simulink model "mini_project_part21"  (R2023b)
settings: Solver=VariableStepAuto  StartTime=0.0  StopTime=1  RelTol=1e-3
libraries: commdigbbndpm3 x2, commchan3 x1, commrandsrc3 x1, commsink2 x1
settings Model: Creator=lx69  LastModifiedBy=xieluxi

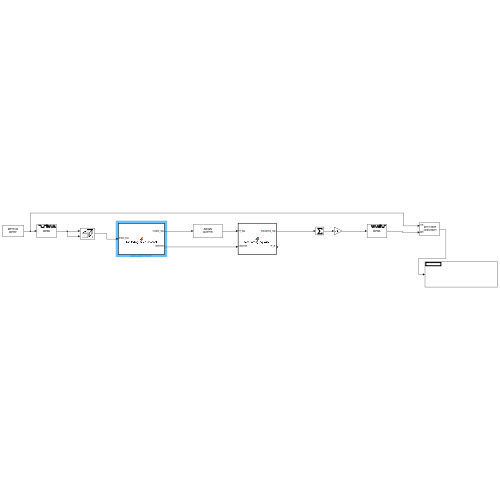
[thumbnail: Simulink's stored preview of the top-level diagram]
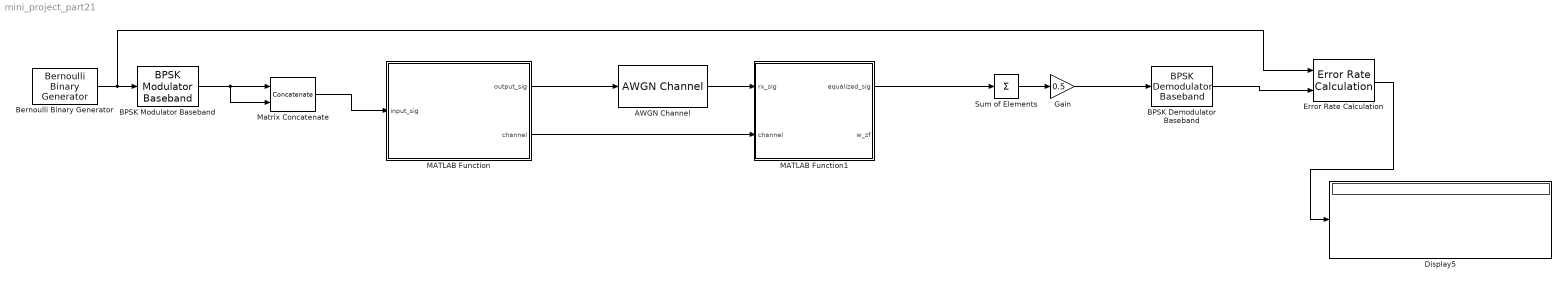
== system mini_project_part21 ==
  AWGN Channel : commchan3/AWGN Channel  LegacyMode=off  NoiseMethod="Signal to noise ratio  (SNR)"  noiseMode="Signal to noise ratio  (SNR)"  EbNo=0  EsNo=10  SNR=0  BitsPerSymbol=1  SignalPower=1  SamplesPerSymbol=1  SymbolPeriod=1  VarianceSource=Parameter  Variance=1  RandomStream=Global stream  Seed=67  SimulateUsing=Code generation
  BPSK Demodulator Baseband : commdigbbndpm3/BPSK Demodulator Baseband  DecType=Hard decision  VarSource=Dialog  Variance=1  Ph=0  outDtype=Inherit via internal rule  derotateFactorWordLen=16  derotateFactorDataTypeStr=Inherit: Same word length as input  derotateFactorLastDataTypeStr=Inherit: Same word length as input
      settings: LibrarySourceBlock=|
      | commhdldigbbndpm/BPSK
      | Demodulator
      | Baseband
  BPSK Modulator Baseband : commdigbbndpm3/BPSK Modulator Baseband  Ph=0  outDtype=double  outWordLen=16  outUDDataType=sfix(16)  outFracLenMode=Best precision  outFracLen=15  outDataTypeStr=double  outLastDataTypeStr=double
  Bernoulli Binary Generator : commrandsrc3/Bernoulli Binary Generator  ProbabilityOfZero=0.5  SeedSource=Auto  Seed=0  SampleTime=0.0001  SamplesPerFrame=1  OutputDataType=double  SimulateUsing=Interpreted execution
  Display5 : Display
  Error Rate Calculation : commsink2/Error Rate Calculation  N=0  st_delay=0  cp_mode=Entire frame  subframe=[]  PMode=Port  WsName=ErrorVec  RsMode2=off  stop=off  numErr=100  maxBits=1e6
      settings: LibrarySourceBlock=|
      | commhdlsink/Error Rate
      | Calculation
  Gain : Gain  Gain=0.5
  MATLAB Function : MATLAB Function  TreatAsAtomicUnit=on
  MATLAB Function1 : MATLAB Function  TreatAsAtomicUnit=on
  Matrix Concatenate : Concatenate  Mode=Multidimensional array
  Sum of Elements : Sum  Inputs=+  CollapseDim=2
  wires:
  Bernoulli Binary Generator/1 -> Error Rate Calculation/1, BPSK Modulator Baseband/1
  BPSK Modulator Baseband/1 -> Matrix Concatenate/2, Matrix Concatenate/1
  Matrix Concatenate/1 -> MATLAB Function/1(input_sig)
  MATLAB Function/1(output_sig) -> AWGN Channel/1
  MATLAB Function/2(channel) -> MATLAB Function1/2(channel)
  AWGN Channel/1 -> MATLAB Function1/1(rx_sig)
  BPSK Demodulator Baseband/1 -> Error Rate Calculation/2
  Error Rate Calculation/1 -> Display5/1
  Gain/1 -> BPSK Demodulator Baseband/1
  MATLAB Function1/1(equalized_sig) -> Sum of Elements/1
  Sum of Elements/1 -> Gain/1

== matlab function mini_project_part21/MATLAB Function1 ==
  data: equalized_sig output; w_zf output; rx_sig input; channel input
function [equalized_sig, w_zf]= zero_forcing_equalizer(rx_sig, channel)
w_zf = pinv(channel'*channel)*channel';
equalized_sig = w_zf*rx_sig;

== matlab function mini_project_part21/MATLAB Function ==
  data: input_sig input; output_sig output; channel output
function [output_sig, channel] = flat_fading_mimo_channel(input_sig)

nTx = 2; nRx = 2;

channel = [1 0.1; 0.1 1] + 1j*[1 0.1; 0.1 1];
output_sig = channel*input_sig;

end
